simulink model "single_phase_three_phase_to_motor"  (R2024b)
settings: Solver=ode3  StartTime=0.0  StopTime=10  FixedStep=10e-6  RelTol=1e-3
model workspace (MAT data in the model file):
  pulse_generator_period = 0.02
libraries: spsIGBTLib x6, spsCurrentMeasurementLib x3, spsVoltageMeasurementLib x3, spsAsynchronousMachineSIUnitsLib x1, spsDCVoltageSourceLib x1, spspowerguiLib x1
settings Model: Creator=Abhijith_Kumble  LastModifiedBy=Abhijith_Kumble

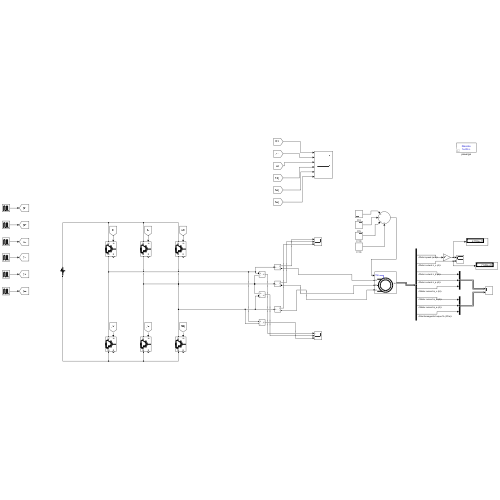
[thumbnail: Simulink's stored preview of the top-level diagram]
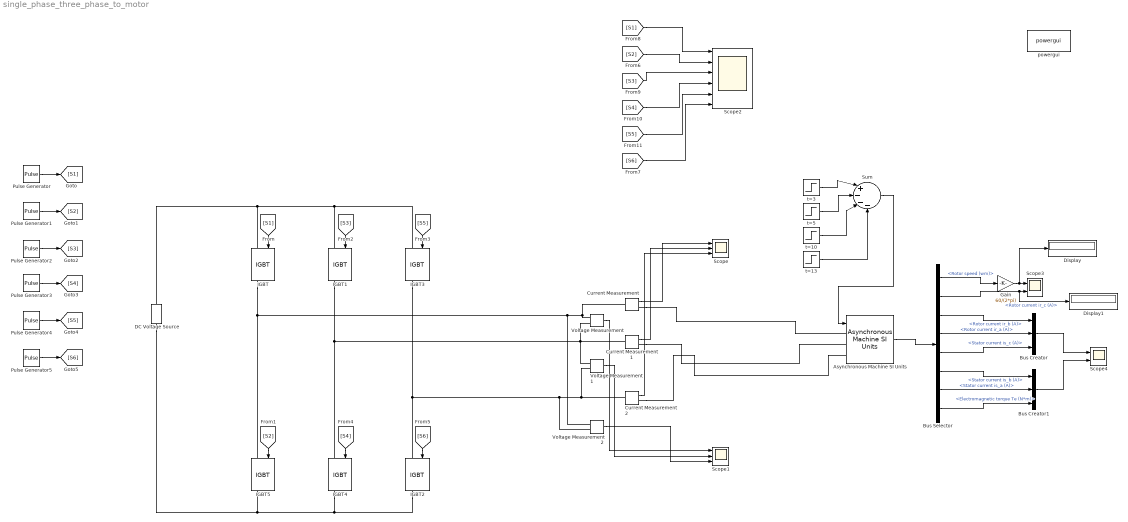
== system single_phase_three_phase_to_motor ==
  Asynchronous Machine SI Units : spsAsynchronousMachineSIUnitsLib/Asynchronous Machine SI Units  RotorType=Squirrel-cage  PresetModel="15:  5.4 HP (4KW)   400 V  50Hz 1430 RPM"  MechanicalLoad=Torque Tm  ShowDetailedParameters=on  ReferenceFrame=Rotor  Units=SI  MeasurementBus=off  NominalParameters=[4000 400 50]  VoltageRatio=1  Stator=[1.405 0.005839]  Rotor=[1.395 0.005839]  Cage1=[0.4155 0.002066]  Cage2=[0.4168 0.0003495]  Lm=0.1722  Mechanical=[0.0131 0.002985 2]  PolePairs=2  InitialConditions=[0 0 0 0 0 0 0 0]  SimulateSaturation=off  Saturation=[14.03593122, 27.81365428, 53.79336849, 72.68890987, 97.98006896, 148.6815601, 215.7428561, 302.9841135, 428.7778367 ; 230, 322, 414, 460, 506, 552, 598, 644, 690]  LoadFlowParameters=1492000  TsPowergui=0  TsBlock=-1  IterativeModel=Trapezoidal non iterative  IterativeDiscreteModel=Trapezoidal non iterative  Pmec=1.492e+006
  Bus Creator : BusCreator  Inputs=3
  Bus Creator1 : BusCreator  Inputs=3
  Bus Selector : BusSelector  OutputSignals=Mechanical.Rotor speed (wm),Rotor measurements.Rotor current ir_c (A),Rotor measurements.Rotor current ir_b (A),Rotor measurements.Rotor current ir_a (A),Stator measurements.Stator current is_c (A),Stator measurements.Stator current is_b (A),Stator measurements.Stator current is_a (A),Mechanical.Electromagnetic torque Te (N*m)
  Current Measurement : spsCurrentMeasurementLib/Current Measurement  PhasorSimulation=off  OutputType=Complex  PSBequivalent=0
  Current Measurement1 : spsCurrentMeasurementLib/Current Measurement  PhasorSimulation=off  OutputType=Complex  PSBequivalent=0
  Current Measurement2 : spsCurrentMeasurementLib/Current Measurement  PhasorSimulation=off  OutputType=Complex  PSBequivalent=0
  DC Voltage Source : spsDCVoltageSourceLib/DC Voltage Source  Amplitude=460/sqrt(3)  Measurements=None
  Display : Display
  Display1 : Display
  Gain : Gain  Gain=60/(2*pi)
  IGBT{,1..5} (6 alike) : spsIGBTLib/IGBT  Ron=0.001  Lon=0  Vf=1  Tf=1e-6  Tt=2e-6  IC=0  Rs=1e5  Cs=inf  Measurements=on
  Pulse Generator : DiscretePulseGenerator  PulseType=Time based  Period=pulse_generator_period  PulseWidth=50
  Pulse Generator1 : DiscretePulseGenerator  PulseType=Time based  Period=pulse_generator_period  PulseWidth=50  PhaseDelay=13.3e-3
  Pulse Generator2 : DiscretePulseGenerator  PulseType=Time based  Period=pulse_generator_period  PulseWidth=50  PhaseDelay=6.67e-3
  Pulse Generator3 : DiscretePulseGenerator  PulseType=Time based  Period=pulse_generator_period  PulseWidth=50
  Pulse Generator4 : DiscretePulseGenerator  PulseType=Time based  Period=pulse_generator_period  PulseWidth=50  PhaseDelay=13.3e-3
  Pulse Generator5 : DiscretePulseGenerator  PulseType=Time based  Period=pulse_generator_period  PulseWidth=50  PhaseDelay=6.67e-3
  Scope : Scope  NumInputPorts=3
  Scope1 : Scope  NumInputPorts=3
  Scope2 : Scope  NumInputPorts=6
  Scope3 : Scope  NumInputPorts=2
  Scope4 : Scope  NumInputPorts=2
  Sum : Sum  Inputs=|+---
  Voltage Measurement : spsVoltageMeasurementLib/Voltage Measurement  PhasorSimulation=off  OutputType=Complex  PSBequivalent=0
  Voltage Measurement1 : spsVoltageMeasurementLib/Voltage Measurement  PhasorSimulation=off  OutputType=Complex  PSBequivalent=0
  Voltage Measurement2 : spsVoltageMeasurementLib/Voltage Measurement  PhasorSimulation=off  OutputType=Complex  PSBequivalent=0
  powergui : spspowerguiLib/powergui  Priority=1  SimulationMode=Discrete  SampleTime=10e-6  frequency=60  Iterations=50  frequencyindice=0  Pbase=100e6  ErrMax=1e-4  UnitsV=kV  UnitsW=MW  buscounter=0  FunctionMessages=off  echomessages=off  EnableUseOfTLC=off  CurrentSourceSwitches=off  DisableSnubberDevices=off  DisableRonSwitches=off  DisableVfSwitches=off  DisplayEquations=off  AutomaticDiscreteSolvers=off  SolverType=Tustin/Backward Euler (TBE)  Interpol=off  ExternalGateDelay=off  methode=off  Ts=100  x0status=blocks  SPID=on  SwTol=0  HookPort=off  NonlinearTolerance=1e-4  nMaxIteration=100  ContinueOnMaxIteration=off  RestoreLinks=warning  ResistiveCurrentMeasurement=off  Frange=[0:2:500]  Ylog=off  Xlog=on  ShowGrid=off  save=off  variable=ZData  structure=0  ZoomFFT=off  StartTime=0.0  cycles=1  DisplayStyle=1  fundamental=60  FreqAxis=off  MaxFrequency=1000  frequencyindicesteady=1  RmsSteady=1  display=off
  t=10 : Step  Time=10  After=6.68  SampleTime=0
  t=13 : Step  Time=13  After=6.68  SampleTime=0
  t=3 : Step  Time=3  After=26.72  SampleTime=0
  t=5 : Step  Time=5  After=13.36  SampleTime=0
  wires:
  Current Measurement/1 -> Scope/1
  Current Measurement1/1 -> Scope/2
  Current Measurement2/1 -> Scope/3
  Voltage Measurement/1 -> Scope1/1
  Voltage Measurement1/1 -> Scope1/2
  Voltage Measurement2/1 -> Scope1/3
  Pulse Generator/1 -> [S1]
  [S1] -> IGBT/1
  [S2] -> IGBT5/1
  [S3] -> IGBT1/1
  [S5] -> IGBT3/1
  [S4] -> IGBT4/1
  [S6] -> IGBT2/1
  Pulse Generator1/1 -> [S2]
  Pulse Generator2/1 -> [S3]
  Pulse Generator4/1 -> [S5]
  Pulse Generator3/1 -> [S4]
  Pulse Generator5/1 -> [S6]
  [S1] -> Scope2/1
  [S2] -> Scope2/2
  [S3] -> Scope2/3
  [S4] -> Scope2/4
  [S5] -> Scope2/5
  [S6] -> Scope2/6
  t=3/1 -> Sum/1
  t=5/1 -> Sum/2
  t=10/1 -> Sum/3
  t=13/1 -> Sum/4
  Sum/1 -> Asynchronous Machine SI Units/1
  Asynchronous Machine SI Units/1 -> Bus Selector/1
  Bus Selector/1 -> Gain/1  "<Rotor speed (wm)>"
  Bus Selector/2 -> Display1/1, Scope3/2  "<Rotor current ir_c (A)>"
  Bus Selector/3 -> Bus Creator/1  "<Rotor current ir_b (A)>"
  Bus Selector/4 -> Bus Creator/2  "<Rotor current ir_a (A)>"
  Bus Selector/5 -> Bus Creator/3  "<Stator current is_c (A)>"
  Bus Selector/6 -> Bus Creator1/1  "<Stator current is_b (A)>"
  Bus Selector/7 -> Bus Creator1/2  "<Stator current is_a (A)>"
  Bus Selector/8 -> Bus Creator1/3  "<Electromagnetic torque Te (N*m)>"
  Bus Creator/1 -> Scope4/1
  Bus Creator1/1 -> Scope4/2
  Gain/1 -> Display/1, Scope3/1
  connections:
  IGBT/RConn1 -- Voltage Measurement2/LConn1 -- Current Measurement/LConn1 -- Voltage Measurement/LConn1 -- IGBT5/LConn1
  IGBT1/RConn1 -- IGBT4/LConn1 -- Voltage Measurement1/LConn1 -- Current Measurement1/LConn1 -- Voltage Measurement/LConn2
  IGBT3/RConn1 -- Voltage Measurement2/LConn2 -- Voltage Measurement1/LConn2 -- Current Measurement2/LConn1 -- IGBT2/LConn1
  DC Voltage Source/RConn1 -- IGBT3/LConn1 -- IGBT1/LConn1 -- IGBT/LConn1
  DC Voltage Source/LConn1 -- IGBT2/RConn1 -- IGBT4/RConn1 -- IGBT5/RConn1
  Current Measurement/RConn1 -- Asynchronous Machine SI Units/LConn1
  Current Measurement2/RConn1 -- Asynchronous Machine SI Units/LConn3
  Current Measurement1/RConn1 -- Asynchronous Machine SI Units/LConn2
